simulink model "d2_pacemaker_rate_adaptive"  (R2024b)
settings: Solver=FixedStepAuto  StartTime=0.0  StopTime=10.0  RelTol=1e-3  EnableMultiTasking=on
undefined symbols (not defined in the file): D0, D1, D10, D11, D12, D13, D2, D3, D4, D5, D6, D7, D8, D9, PTA0, PTA1, PTA2, PTB23, PTB9, PTC16, PTC17, PTC2, PTC3, PTC4, PTD0, PTD1, PTD2, PTD3
libraries: frdmk64flib x16, simulink x1
settings Model: ExtModeTrigDuration=5  Creator=cakes  LastModifiedBy=ryans
settings OptimizationCC: EnhancedBackFolding=on  PassReuseOutputArgsAs=Individual arguments  ZeroExternalMemoryAtStartup=off  ZeroInternalMemoryAtStartup=off  MaxStackSize=64  OptimizeBlockOrder=speed  DifferentSizesBufferReuse=on  OptimizationCustomize=off  EfficientTunableParamExpr=on
settings DebuggingCC: ParameterTunabilityLossMsg=error
settings HardwareCC: ProdBitPerPointer=32  ProdBitPerSizeT=32  ProdBitPerPtrDiffT=32  ProdLargestAtomicInteger=Long  ProdLargestAtomicFloat=Double  ProdWordSize=32  ProdHWDeviceType=ARM Compatible->ARM Cortex
settings SFSimCC: MATLABDynamicMemAlloc=off
settings RTWCC: Description=Embedded Coder  SystemTargetFile=ert.tlc  HardwareBoard=NXP FRDM-K64F  TLCOptions="-aInlineSetEventsForThisBaseRateFcn=TLC_FALSE -aSuppressMultiTaskScheduler=TLC_FALSE  -aRateBasedStepFcn=0"  TemplateMakefile=ert_default_tmf  Toolchain=GNU Tools for ARM Embedded Processors  GPUComputeCapability=3.5
settings CodeAppCC: ForceParamTrailComments=on  IgnoreCustomStorageClasses=off  OperatorAnnotations=on  SimulinkDataObjDesc=on  SFDataObjDesc=on  InsertBlockDesc=on
settings ERTTargetCC: ExtModeTransport=4  ExtModeMexFile=sendToCommService  InlinedParameterPlacement=Hierarchical  DynamicArrayContainerType=coder::array

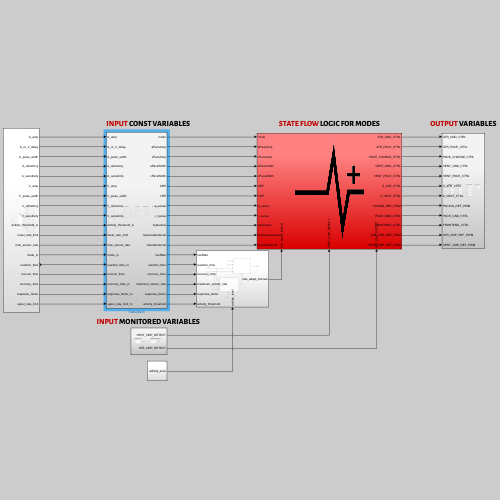
[thumbnail: Simulink's stored preview of the top-level diagram]
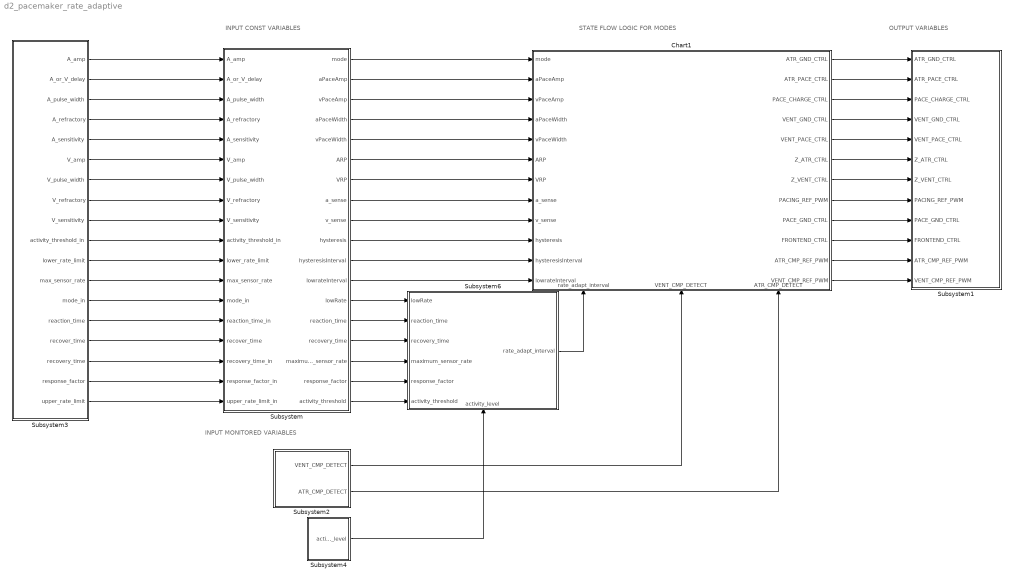
== system d2_pacemaker_rate_adaptive ==
  note: STATE FLOW LOGIC FOR MODES
  note: INPUT CONST VARIABLES
  note: OUTPUT VARIABLES
  note: INPUT MONITORED VARIABLES
  Chart1 : Stateflow chart  TreatAsAtomicUnit=on
      settings: PortSchema="{\"entries\":[{\"content\":{\"sides\":[{\"content\":{\"connectorIds\":[\"In12\",\"In3\",\"In4\",\"In5\",\"In6\",\"In7\",\"In8\",\"In10\",\"In11\",\"In14\",\"In13\",\"In9\"]},\"type\":\"ConnectorPlacement.EquallySpacedRectSide\",\"uuid\":\"0645b224-ea0f-4252-ab3f-59541b69d578\"},{\"content\":{\"connectorIds\":[\"Out1\",\"Out2\",\"Out3\",\"Out4\",\"Out5\",\"Out6\",\"Out7\",\"Out8\",\"Out9\",\"Out10\",\"Out12\",\"Out11\"],\"side\":\"RIGHT\"},\"type\":\"ConnectorPlacement.EquallySpacedRectSide\",\"uuid\":\"774839c9-1eb4-4ab6-be6e-099c2bb8a485\"},{\"content\":{\"side\":\"TOP\"},\"type\":\"ConnectorPlacement.EquallySpacedRectSide\",\"uuid\":\"6cb60565-1780-4b9d-884d-75d2ba8c5024\"},{\"content\":{\"connectorIds\":[\"In15\",\"In1\",\"In2\"],\"side\":\"BOTTOM\"},\"type\":\"ConnectorPlacement.EquallySpacedRectSide\",\"uuid\":\"cb44bc08-16a9-4dba-a42a-7ec56f3e5fd4\"}]},\"type\":\"ConnectorPlacement.EquallySpacedConnector\",\"uuid\":\"755e29d5-bc4e-404e-b866-950d5e4fdc89\"}],\"packageUris\":[\"http://schema.mathworks.com/mf0/Connector/R2020b\"],\"version\":\"1.0\"}"
  Subsystem : Subsystem
  Subsystem1 : Subsystem
  Subsystem2 : Subsystem
  Subsystem3 : Subsystem
  Subsystem4 : Subsystem
  Subsystem6 : Subsystem
      settings: PortSchema="{\"entries\":[{\"content\":{\"sides\":[{\"content\":{\"connectorIds\":[\"In1\",\"In2\",\"In3\",\"In4\",\"In5\",\"In6\"]},\"type\":\"ConnectorPlacement.EquallySpacedRectSide\",\"uuid\":\"7c382d61-8e28-44bb-b5ec-cecd61deb93c\"},{\"content\":{\"connectorIds\":[\"Out1\"],\"side\":\"RIGHT\"},\"type\":\"ConnectorPlacement.EquallySpacedRectSide\",\"uuid\":\"ba607a06-9c8b-48b6-beed-6548638f0809\"},{\"content\":{\"side\":\"TOP\"},\"type\":\"ConnectorPlacement.EquallySpacedRectSide\",\"uuid\":\"ca821f3b-307e-4b9c-9eb8-988783752b3e\"},{\"content\":{\"connectorIds\":[\"In7\"],\"side\":\"BOTTOM\"},\"type\":\"ConnectorPlacement.EquallySpacedRectSide\",\"uuid\":\"dfc7f063-00f5-44f6-92e9-8ee3160489ca\"}]},\"type\":\"ConnectorPlacement.EquallySpacedConnector\",\"uuid\":\"0907d1dd-ec4b-4750-8c68-e4bda9ce45d8\"}],\"packageUris\":[\"http://schema.mathworks.com/mf0/Connector/R2020b\"],\"version\":\"1.0\"}"
  wires:
  Subsystem/2(aPaceAmp) -> Chart1/3(aPaceAmp)
  Subsystem/3(vPaceAmp) -> Chart1/4(vPaceAmp)
  Subsystem/4(aPaceWidth) -> Chart1/5(aPaceWidth)
  Subsystem/5(vPaceWidth) -> Chart1/6(vPaceWidth)
  Subsystem/6(ARP) -> Chart1/7(ARP)
  Subsystem/7(VRP) -> Chart1/8(VRP)
  Subsystem/12(lowrateInterval) -> Chart1/9(lowrateInterval)
  Subsystem/1(mode) -> Chart1/12(mode)
  Chart1/1(ATR_GND_CTRL) -> Subsystem1/1(ATR_GND_CTRL)
  Chart1/2(ATR_PACE_CTRL) -> Subsystem1/2(ATR_PACE_CTRL)
  Chart1/3(PACE_CHARGE_CTRL) -> Subsystem1/3(PACE_CHARGE_CTRL)
  Chart1/4(VENT_GND_CTRL) -> Subsystem1/4(VENT_GND_CTRL)
  Chart1/5(VENT_PACE_CTRL) -> Subsystem1/5(VENT_PACE_CTRL)
  Chart1/6(Z_ATR_CTRL) -> Subsystem1/6(Z_ATR_CTRL)
  Subsystem2/1(VENT_CMP_DETECT) -> Chart1/1(VENT_CMP_DETECT)
  Chart1/9(PACE_GND_CTRL) -> Subsystem1/9(PACE_GND_CTRL)
  Subsystem/8(a_sense) -> Chart1/10(a_sense)
  Subsystem/9(v_sense) -> Chart1/11(v_sense)
  Chart1/10(FRONTEND_CTRL) -> Subsystem1/10(FRONTEND_CTRL)
  Chart1/11(VENT_CMP_REF_PWM) -> Subsystem1/12(VENT_CMP_REF_PWM)
  Chart1/7(Z_VENT_CTRL) -> Subsystem1/7(Z_VENT_CTRL)
  Chart1/8(PACING_REF_PWM) -> Subsystem1/8(PACING_REF_PWM)
  Chart1/12(ATR_CMP_REF_PWM) -> Subsystem1/11(ATR_CMP_REF_PWM)
  Subsystem2/2(ATR_CMP_DETECT) -> Chart1/2(ATR_CMP_DETECT)
  Subsystem/10(hysteresis) -> Chart1/14(hysteresis)
  Subsystem/11(hysteresisInterval) -> Chart1/13(hysteresisInterval)
  Subsystem/17(response_factor) -> Subsystem6/5(response_factor)
  Subsystem/16(maximum_sensor_rate) -> Subsystem6/4(maximum_sensor_rate)
  Subsystem/13(lowRate) -> Subsystem6/1(lowRate)
  Subsystem/14(reaction_time) -> Subsystem6/2(reaction_time)
  Subsystem/15(recovery_time) -> Subsystem6/3(recovery_time)
  Subsystem/18(activity_threshold) -> Subsystem6/6(activity_threshold)
  Subsystem6/1(rate_adapt_interval) -> Chart1/15(rate_adapt_interval)
  Subsystem4/1(activity_level) -> Subsystem6/7(activity_level)
  Subsystem3/1(A_amp) -> Subsystem/1(A_amp)
  Subsystem3/3(A_pulse_width) -> Subsystem/3(A_pulse_width)
  Subsystem3/4(A_refractory) -> Subsystem/4(A_refractory)
  Subsystem3/5(A_sensitivity) -> Subsystem/5(A_sensitivity)
  Subsystem3/6(V_amp) -> Subsystem/6(V_amp)
  Subsystem3/7(V_pulse_width) -> Subsystem/7(V_pulse_width)
  Subsystem3/8(V_refractory) -> Subsystem/8(V_refractory)
  Subsystem3/9(V_sensitivity) -> Subsystem/9(V_sensitivity)
  Subsystem3/11(lower_rate_limit) -> Subsystem/11(lower_rate_limit)
  Subsystem3/12(max_sensor_rate) -> Subsystem/12(max_sensor_rate)
  Subsystem3/13(mode_in) -> Subsystem/13(mode_in)
  Subsystem3/15(recover_time) -> Subsystem/15(recover_time)
  Subsystem3/16(recovery_time) -> Subsystem/16(recovery_time_in)
  Subsystem3/17(response_factor) -> Subsystem/17(response_factor_in)
  Subsystem3/18(upper_rate_limit) -> Subsystem/18(upper_rate_limit_in)
  Subsystem3/2(A_or_V_delay) -> Subsystem/2(A_or_V_delay)
  Subsystem3/10(activity_threshold_in) -> Subsystem/10(activity_threshold_in)
  Subsystem3/14(reaction_time) -> Subsystem/14(reaction_time_in)

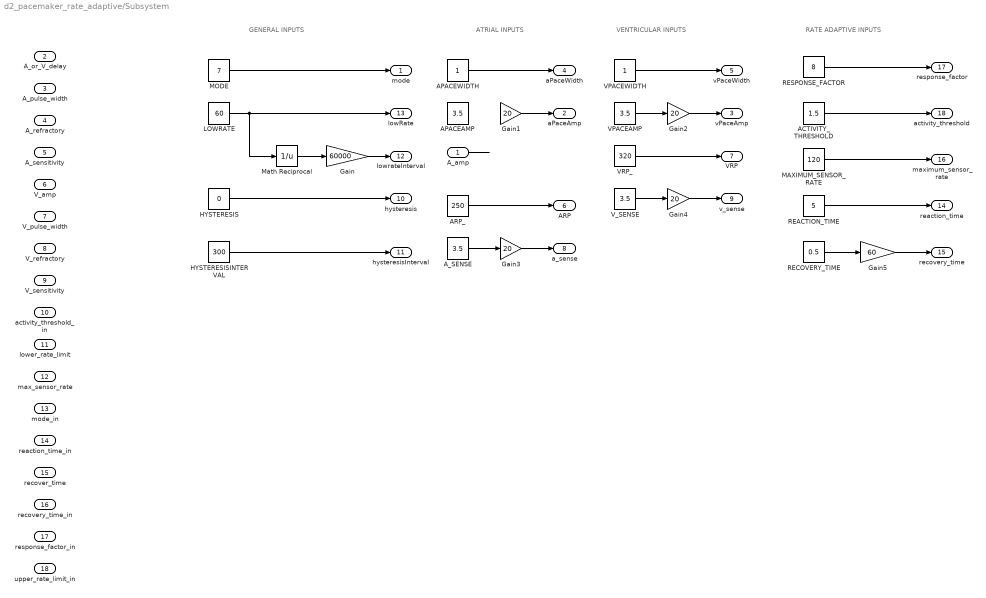
== system d2_pacemaker_rate_adaptive/Subsystem ==
  note: GENERAL INPUTS
  note: ATRIAL INPUTS
  note: VENTRICULAR INPUTS
  note: RATE ADAPTIVE INPUTS
  A_amp : Inport  OutDataTypeStr=single
  A_or_V_delay : Inport  Port=2
  A_pulse_width : Inport  Port=3
  A_refractory : Inport  Port=4
  A_sensitivity : Inport  Port=5
  V_amp : Inport  Port=6
  V_pulse_width : Inport  Port=7
  V_refractory : Inport  Port=8
  V_sensitivity : Inport  Port=9
  activity_threshold_in : Inport  Port=10
  lower_rate_limit : Inport  Port=11
  max_sensor_rate : Inport  Port=12
  mode_in : Inport  Port=13
  reaction_time_in : Inport  Port=14
  recover_time : Inport  Port=15
  recovery_time_in : Inport  Port=16
  response_factor_in : Inport  Port=17
  upper_rate_limit_in : Inport  Port=18
  ACTIVITY_THRESHOLD : Constant  Value=1.5
  APACEAMP : Constant  Value=3.5
  APACEWIDTH : Constant
  ARP_ : Constant  Value=250
  A_SENSE : Constant  Value=3.5
  Gain : Gain  Gain=60000
  Gain{1..4} (4 alike) : Gain  Gain=20
  Gain5 : Gain  Gain=60
  HYSTERESIS : Constant  Value=0
  HYSTERESISINTERVAL : Constant  Value=300
  LOWRATE : Constant  Value=60
  MAXIMUM_SENSOR_RATE : Constant  Value=120
  MODE : Constant  Value=7
  Math Reciprocal : Math  Operator=reciprocal  SignedPower=on
  REACTION_TIME : Constant  Value=5
  RECOVERY_TIME : Constant  Value=0.5
  RESPONSE_FACTOR : Constant  Value=8
  VPACEAMP : Constant  Value=3.5
  VPACEWIDTH : Constant
  VRP_ : Constant  Value=320
  V_SENSE : Constant  Value=3.5
  mode : Outport
  aPaceAmp : Outport  Port=2
  vPaceAmp : Outport  Port=3
  aPaceWidth : Outport  Port=4
  vPaceWidth : Outport  Port=5
  ARP : Outport  Port=6
  VRP : Outport  Port=7
  a_sense : Outport  Port=8
  v_sense : Outport  Port=9
  hysteresis : Outport  Port=10
  hysteresisInterval : Outport  Port=11
  lowrateInterval : Outport  Port=12
  lowRate : Outport  Port=13
  reaction_time : Outport  Port=14
  recovery_time : Outport  Port=15
  maximum_sensor_rate : Outport  Port=16
  response_factor : Outport  Port=17
  activity_threshold : Outport  Port=18
  wires:
  APACEWIDTH/1 -> aPaceWidth/1
  VPACEWIDTH/1 -> vPaceWidth/1
  MODE/1 -> mode/1
  ARP_/1 -> ARP/1
  VRP_/1 -> VRP/1
  HYSTERESIS/1 -> hysteresis/1
  HYSTERESISINTERVAL/1 -> hysteresisInterval/1
  LOWRATE/1 -> lowRate/1, Math Reciprocal/1
  Math Reciprocal/1 -> Gain/1
  Gain/1 -> lowrateInterval/1
  Gain1/1 -> aPaceAmp/1
  VPACEAMP/1 -> Gain2/1
  Gain2/1 -> vPaceAmp/1
  A_SENSE/1 -> Gain3/1
  V_SENSE/1 -> Gain4/1
  Gain4/1 -> v_sense/1
  Gain3/1 -> a_sense/1
  RESPONSE_FACTOR/1 -> response_factor/1
  ACTIVITY_THRESHOLD/1 -> activity_threshold/1
  RECOVERY_TIME/1 -> Gain5/1
  Gain5/1 -> recovery_time/1
  REACTION_TIME/1 -> reaction_time/1
  MAXIMUM_SENSOR_RATE/1 -> maximum_sensor_rate/1
  A_amp/1 -> ?

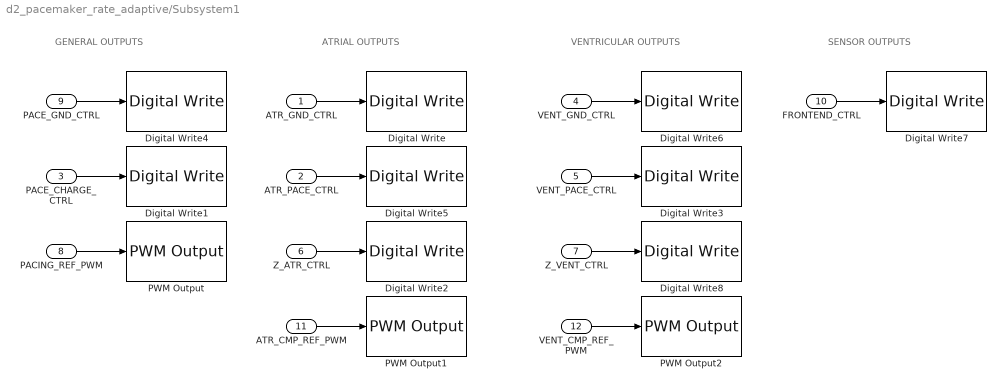
== system d2_pacemaker_rate_adaptive/Subsystem1 ==
  note: ATRIAL OUTPUTS
  note: GENERAL OUTPUTS
  note: VENTRICULAR OUTPUTS
  note: SENSOR OUTPUTS
  ATR_GND_CTRL : Inport
  ATR_PACE_CTRL : Inport  Port=2
  PACE_CHARGE_CTRL : Inport  Port=3
  VENT_GND_CTRL : Inport  Port=4
  VENT_PACE_CTRL : Inport  Port=5
  Z_ATR_CTRL : Inport  Port=6
  Z_VENT_CTRL : Inport  Port=7
  PACING_REF_PWM : Inport  Port=8
  PACE_GND_CTRL : Inport  Port=9
  FRONTEND_CTRL : Inport  Port=10
  ATR_CMP_REF_PWM : Inport  Port=11
  VENT_CMP_REF_PWM : Inport  Port=12
  Digital Write : frdmk64flib/Digital Write  Whichpin=PTD2 (D11)
  Digital Write1 : frdmk64flib/Digital Write  Whichpin=PTB9 (D2)
  Digital Write2 : frdmk64flib/Digital Write  Whichpin=PTB23 (D4)
  Digital Write3 : frdmk64flib/Digital Write  Whichpin=PTC4 (D9)
  Digital Write4 : frdmk64flib/Digital Write  Whichpin=PTD0 (D10)
  Digital Write5 : frdmk64flib/Digital Write  Whichpin=PTA0 (D8)
  Digital Write6 : frdmk64flib/Digital Write  Whichpin=PTD3 (D12)
  Digital Write7 : frdmk64flib/Digital Write  Whichpin=PTD1 (D13)
  Digital Write8 : frdmk64flib/Digital Write  Whichpin=PTC3 (D7)
  PWM Output : frdmk64flib/PWM Output  Whichpin=PTA2 (D5)  InitialFrequency=2000  InitialDutyCycle=0
  PWM Output1 : frdmk64flib/PWM Output  Whichpin=PTC2 (D6)  InitialFrequency=2000  InitialDutyCycle=0
  PWM Output2 : frdmk64flib/PWM Output  Whichpin=PTA1 (D3)  InitialFrequency=2000  InitialDutyCycle=0
  wires:
  PACING_REF_PWM/1 -> PWM Output/1
  Z_ATR_CTRL/1 -> Digital Write2/1
  PACE_CHARGE_CTRL/1 -> Digital Write1/1
  ATR_PACE_CTRL/1 -> Digital Write5/1
  ATR_GND_CTRL/1 -> Digital Write/1
  VENT_PACE_CTRL/1 -> Digital Write3/1
  VENT_GND_CTRL/1 -> Digital Write6/1
  FRONTEND_CTRL/1 -> Digital Write7/1
  Z_VENT_CTRL/1 -> Digital Write8/1
  PACE_GND_CTRL/1 -> Digital Write4/1
  ATR_CMP_REF_PWM/1 -> PWM Output1/1
  VENT_CMP_REF_PWM/1 -> PWM Output2/1

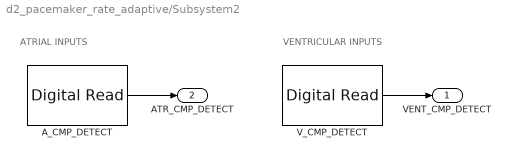
== system d2_pacemaker_rate_adaptive/Subsystem2 ==
  note: ATRIAL INPUTS
  note: VENTRICULAR INPUTS
  A_CMP_DETECT : frdmk64flib/Digital Read  Whichpin=PTC16 (D0)  SampleTime=0.01
  V_CMP_DETECT : frdmk64flib/Digital Read  Whichpin=PTC17 (D1)  SampleTime=0.01
  VENT_CMP_DETECT : Outport
  ATR_CMP_DETECT : Outport  Port=2
  wires:
  V_CMP_DETECT/1 -> VENT_CMP_DETECT/1
  A_CMP_DETECT/1 -> ATR_CMP_DETECT/1

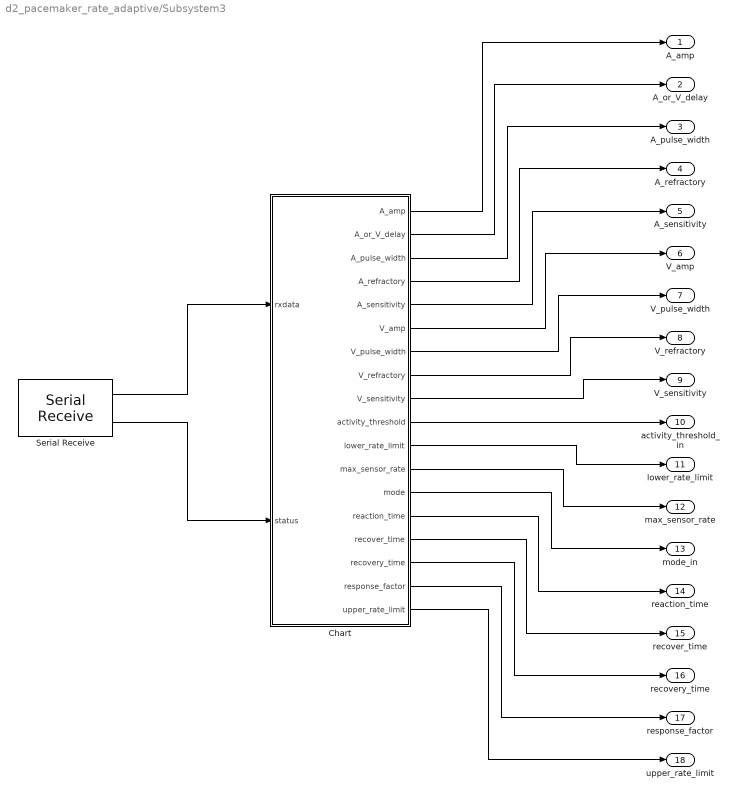
== system d2_pacemaker_rate_adaptive/Subsystem3 ==
  Chart : Stateflow chart  TreatAsAtomicUnit=on
  Serial Receive : frdmk64flib/Serial Receive  SCIModule=0  Baudrate=uint32(9600)  Parity=None  StopBits=1  HardwareFlowControl=None  ByteOrder=LittleEndian  DataType=uint8  DataLength=10  BlockingMode=off  OutputStatus=on  SampleTime=0.1
  A_amp : Outport
  A_or_V_delay : Outport  Port=2
  A_pulse_width : Outport  Port=3
  A_refractory : Outport  Port=4
  A_sensitivity : Outport  Port=5
  V_amp : Outport  Port=6
  V_pulse_width : Outport  Port=7
  V_refractory : Outport  Port=8
  V_sensitivity : Outport  Port=9
  activity_threshold_in : Outport  Port=10
  lower_rate_limit : Outport  Port=11
  max_sensor_rate : Outport  Port=12
  mode_in : Outport  Port=13
  reaction_time : Outport  Port=14
  recover_time : Outport  Port=15
  recovery_time : Outport  Port=16
  response_factor : Outport  Port=17
  upper_rate_limit : Outport  Port=18
  wires:
  Serial Receive/1 -> Chart/1(rxdata)
  Serial Receive/2 -> Chart/2(status)
  Chart/1(A_amp) -> A_amp/1
  Chart/2(A_or_V_delay) -> A_or_V_delay/1
  Chart/3(A_pulse_width) -> A_pulse_width/1
  Chart/4(A_refractory) -> A_refractory/1
  Chart/5(A_sensitivity) -> A_sensitivity/1
  Chart/6(V_amp) -> V_amp/1
  Chart/7(V_pulse_width) -> V_pulse_width/1
  Chart/8(V_refractory) -> V_refractory/1
  Chart/9(V_sensitivity) -> V_sensitivity/1
  Chart/10(activity_threshold) -> activity_threshold_in/1
  Chart/11(lower_rate_limit) -> lower_rate_limit/1
  Chart/12(max_sensor_rate) -> max_sensor_rate/1
  Chart/13(mode) -> mode_in/1
  Chart/14(reaction_time) -> reaction_time/1
  Chart/15(recover_time) -> recover_time/1
  Chart/16(recovery_time) -> recovery_time/1
  Chart/17(response_factor) -> response_factor/1
  Chart/18(upper_rate_limit) -> upper_rate_limit/1

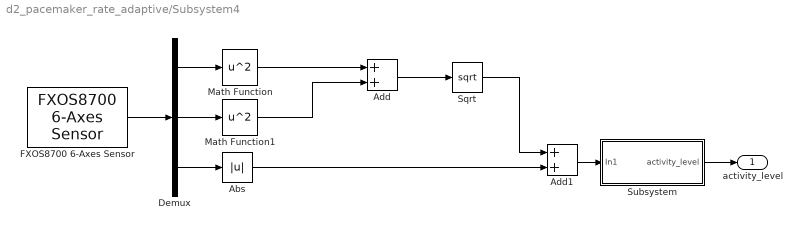
== system d2_pacemaker_rate_adaptive/Subsystem4 ==
  Abs : Abs  SaturateOnIntegerOverflow=off
  Add : Sum
  Add1 : Sum
  Demux : Demux  Outputs=3
  FXOS8700 6-Axes Sensor : frdmk64flib/FXOS8700 6-Axes Sensor  Activesensor=Accelerometer only  ODR=50Hz  HybridODR=400Hz  Accelfullrange=-4g to +4g  SampleTime=0.01
  Math Function : Math  Operator=square
  Math Function1 : Math  Operator=square
  Sqrt : Sqrt
  Subsystem : Subsystem
  activity_level : Outport
  wires:
  Demux/2 -> Math Function1/1
  Math Function/1 -> Add/1
  Math Function1/1 -> Add/2
  Sqrt/1 -> Add1/1
  Abs/1 -> Add1/2
  Add/1 -> Sqrt/1
  Demux/1 -> Math Function/1
  Demux/3 -> Abs/1
  FXOS8700 6-Axes Sensor/1 -> Demux/1
  Add1/1 -> Subsystem/1(In1)
  Subsystem/1(activity_level) -> activity_level/1

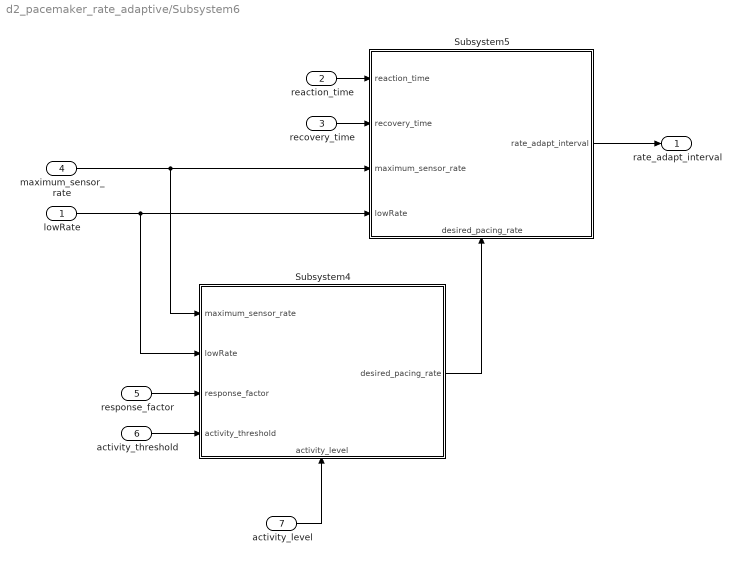
== system d2_pacemaker_rate_adaptive/Subsystem6 ==
  lowRate : Inport
  reaction_time : Inport  Port=2
  recovery_time : Inport  Port=3
  maximum_sensor_rate : Inport  Port=4
  response_factor : Inport  Port=5
  activity_threshold : Inport  Port=6
  activity_level : Inport  Port=7
  Subsystem4 : Subsystem
      settings: PortSchema="{\"entries\":[{\"content\":{\"sides\":[{\"content\":{\"connectorIds\":[\"In1\",\"In2\",\"In3\",\"In4\"]},\"type\":\"ConnectorPlacement.EquallySpacedRectSide\",\"uuid\":\"79bc3fb3-9fea-4441-ae48-8f2cb8dc5d6d\"},{\"content\":{\"connectorIds\":[\"Out1\"],\"side\":\"RIGHT\"},\"type\":\"ConnectorPlacement.EquallySpacedRectSide\",\"uuid\":\"8e25f63d-7a7f-4a30-9d51-ff4e93a9aa99\"},{\"content\":{\"side\":\"TOP\"},\"type\":\"ConnectorPlacement.EquallySpacedRectSide\",\"uuid\":\"e07be596-e475-4181-9b08-2e1f9ea03076\"},{\"content\":{\"connectorIds\":[\"In5\"],\"side\":\"BOTTOM\"},\"type\":\"ConnectorPlacement.EquallySpacedRectSide\",\"uuid\":\"45319594-5d17-4fc8-9d4a-dc1aca31fcf6\"}]},\"type\":\"ConnectorPlacement.EquallySpacedConnector\",\"uuid\":\"3beff34e-2a6c-47b3-9523-1069d662617f\"}],\"packageUris\":[\"http://schema.mathworks.com/mf0/Connector/R2020b\"],\"version\":\"1.0\"}"
  Subsystem5 : Subsystem
      settings: PortSchema="{\"entries\":[{\"content\":{\"sides\":[{\"content\":{\"connectorIds\":[\"In1\",\"In2\",\"In3\",\"In4\"]},\"type\":\"ConnectorPlacement.EquallySpacedRectSide\",\"uuid\":\"79bc3fb3-9fea-4441-ae48-8f2cb8dc5d6d\"},{\"content\":{\"connectorIds\":[\"Out1\"],\"side\":\"RIGHT\"},\"type\":\"ConnectorPlacement.EquallySpacedRectSide\",\"uuid\":\"8e25f63d-7a7f-4a30-9d51-ff4e93a9aa99\"},{\"content\":{\"side\":\"TOP\"},\"type\":\"ConnectorPlacement.EquallySpacedRectSide\",\"uuid\":\"e07be596-e475-4181-9b08-2e1f9ea03076\"},{\"content\":{\"connectorIds\":[\"In5\"],\"side\":\"BOTTOM\"},\"type\":\"ConnectorPlacement.EquallySpacedRectSide\",\"uuid\":\"37a509d1-15c0-445b-9b56-eefd17d0fdfa\"}]},\"type\":\"ConnectorPlacement.EquallySpacedConnector\",\"uuid\":\"3beff34e-2a6c-47b3-9523-1069d662617f\"}],\"packageUris\":[\"http://schema.mathworks.com/mf0/Connector/R2020b\"],\"version\":\"1.0\"}"
  rate_adapt_interval : Outport
  wires:
  Subsystem5/1(rate_adapt_interval) -> rate_adapt_interval/1
  reaction_time/1 -> Subsystem5/1(reaction_time)
  recovery_time/1 -> Subsystem5/2(recovery_time)
  Subsystem4/1(desired_pacing_rate) -> Subsystem5/5(desired_pacing_rate)
  maximum_sensor_rate/1 -> Subsystem4/1(maximum_sensor_rate), Subsystem5/3(maximum_sensor_rate)
  lowRate/1 -> Subsystem4/2(lowRate), Subsystem5/4(lowRate)
  activity_threshold/1 -> Subsystem4/4(activity_threshold)
  response_factor/1 -> Subsystem4/3(response_factor)
  activity_level/1 -> Subsystem4/5(activity_level)

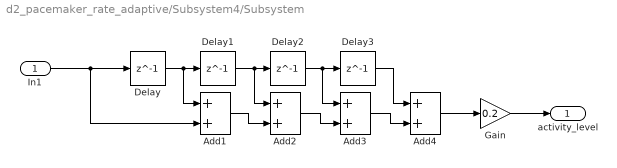
== system d2_pacemaker_rate_adaptive/Subsystem4/Subsystem ==
  In1 : Inport
  Add{1..4} (4 alike) : Sum
  Delay{,1..3} (4 alike) : Delay  DelayLength=1
  Gain : Gain  Gain=0.2
  activity_level : Outport
  wires:
  Delay/1 -> Add1/1, Delay1/1
  Delay1/1 -> Add2/1, Delay2/1
  Delay2/1 -> Add3/1, Delay3/1
  In1/1 -> Delay/1, Add1/2
  Add1/1 -> Add2/2
  Add4/1 -> Gain/1
  Add2/1 -> Add3/2
  Add3/1 -> Add4/2
  Delay3/1 -> Add4/1
  Gain/1 -> activity_level/1

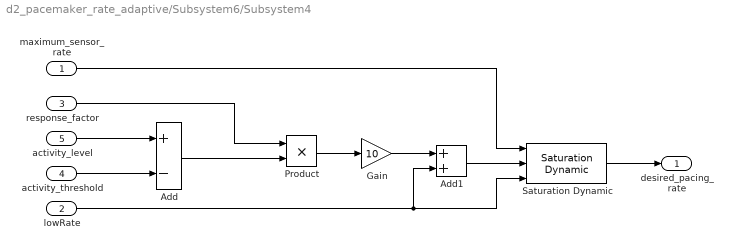
== system d2_pacemaker_rate_adaptive/Subsystem6/Subsystem4 ==
  maximum_sensor_rate : Inport
  lowRate : Inport  Port=2
  response_factor : Inport  Port=3
  activity_threshold : Inport  Port=4
  activity_level : Inport  Port=5
  Add : Sum  Inputs=+-
  Add1 : Sum
  Gain : Gain  Gain=10
  Product : Product
  Saturation Dynamic : simulink/Discontinuities/Saturation Dynamic  OutMin=[]  OutMax=[]  OutDataTypeStr=Inherit: Same as second input  OutDataType=fixdt(1, 16)  OutScaling=2^-10  DoSatur=off
  desired_pacing_rate : Outport
  wires:
  activity_level/1 -> Add/1
  activity_threshold/1 -> Add/2
  Add/1 -> Product/2
  response_factor/1 -> Product/1
  Gain/1 -> Add1/1
  Product/1 -> Gain/1
  lowRate/1 -> Saturation Dynamic/3, Add1/2
  Add1/1 -> Saturation Dynamic/2
  maximum_sensor_rate/1 -> Saturation Dynamic/1
  Saturation Dynamic/1 -> desired_pacing_rate/1

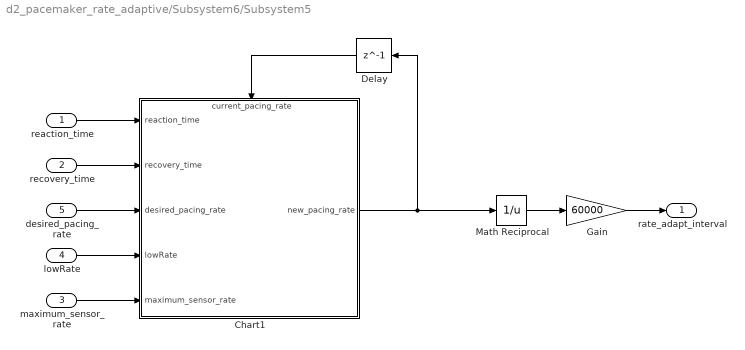
== system d2_pacemaker_rate_adaptive/Subsystem6/Subsystem5 ==
  reaction_time : Inport
  recovery_time : Inport  Port=2
  maximum_sensor_rate : Inport  Port=3
  lowRate : Inport  Port=4
  desired_pacing_rate : Inport  Port=5
  Chart1 : Stateflow chart  TreatAsAtomicUnit=on
      settings: PortSchema="{\"entries\":[{\"content\":{\"sides\":[{\"content\":{\"connectorIds\":[\"In2\",\"In3\",\"In4\",\"In5\",\"In6\"]},\"type\":\"ConnectorPlacement.EquallySpacedRectSide\",\"uuid\":\"06a0217b-4288-43b0-8932-705b4d4ece1e\"},{\"content\":{\"connectorIds\":[\"Out1\"],\"side\":\"RIGHT\"},\"type\":\"ConnectorPlacement.EquallySpacedRectSide\",\"uuid\":\"c8eefe2e-d095-40c8-acb0-aebaf19a9365\"},{\"content\":{\"connectorIds\":[\"In1\"],\"side\":\"TOP\"},\"type\":\"ConnectorPlacement.EquallySpacedRectSide\",\"uuid\":\"128ffed5-e0e5-4f4f-9131-f15ad41e2462\"},{\"content\":{\"side\":\"BOTTOM\"},\"type\":\"ConnectorPlacement.EquallySpacedRectSide\",\"uuid\":\"a7475944-bf84-45a0-8219-ddf2a50d7d23\"}]},\"type\":\"ConnectorPlacement.EquallySpacedConnector\",\"uuid\":\"00626f3d-df19-4fc7-9d9d-9a6ae210b908\"}],\"packageUris\":[\"http://schema.mathworks.com/mf0/Connector/R2020b\"],\"version\":\"1.0\"}"
  Delay : Delay  DelayLength=1  InitialCondition=0
  Gain : Gain  Gain=60000
  Math Reciprocal : Math  Operator=reciprocal  SignedPower=on
  rate_adapt_interval : Outport
  wires:
  Chart1/1(new_pacing_rate) -> Delay/1, Math Reciprocal/1
  Math Reciprocal/1 -> Gain/1
  Gain/1 -> rate_adapt_interval/1
  reaction_time/1 -> Chart1/2(reaction_time)
  Delay/1 -> Chart1/1(current_pacing_rate)
  maximum_sensor_rate/1 -> Chart1/6(maximum_sensor_rate)
  recovery_time/1 -> Chart1/3(recovery_time)
  lowRate/1 -> Chart1/5(lowRate)
  desired_pacing_rate/1 -> Chart1/4(desired_pacing_rate)

== stateflow chart d2_pacemaker_rate_adaptive/Chart1 ==
  settings: sampleTime=0.001
  state INIT
    entry:
    %inital state, reset variables when mode change
    PACE_CHARGE_CTRL = 0;
    ATR_PACE_CTRL = 0;
    ATR_GND_CTRL = 0;
    VENT_PACE_CTRL=0;
    VENT_GND_CTRL=0;
    Z_ATR_CTRL = 0;
    Z_VENT_CTRL=0;
    PACE_GND_CTRL=0;
    PACING_REF_PWM=0;
    PACE_CHARGE_CTRL=0;
    FRONTEND_CTRL =0;
    VENT_CMP_REF_PWM = v_sense;
    ATR_CMP_REF_PWM = a_sense;
    note: MODE
        | NUMBER
        |
        | AOO
        | 0
        |
        | VOO
        | 1
        |
        | AAI
        | 2
        |
        | VVI
        | 3
  state AOO
    state AOO_Charging
      %charging capacitor
      entry:
      PACING_REF_PWM = aPaceAmp;
      PACE_GND_CTRL = 1;
      Z_ATR_CTRL = 0;
      ATR_PACE_CTRL = 0;
      PACE_CHARGE_CTRL = 1;
      ATR_GND_CTRL = 1;
    state AOO_Pacing
      %discharging
      entry:
      Z_ATR_CTRL = 1;
      PACE_CHARGE_CTRL = 0;
      ATR_GND_CTRL = 0;
      ATR_PACE_CTRL = 1;
    (default) -> AOO_Charging
    AOO_Charging -> AOO_Pacing : after(lowrateInterval - aPaceWidth, msec)
    AOO_Pacing -> AOO_Charging : after(aPaceWidth, msec)
  state VOO
    state VOO_Charging
      %charging capacitor
      entry:
      PACING_REF_PWM = vPaceAmp;
      PACE_GND_CTRL = 1;
      Z_VENT_CTRL = 0;
      VENT_PACE_CTRL = 0;
      PACE_CHARGE_CTRL = 1;
      VENT_GND_CTRL = 1;
    state VOO_Pacing
      %discharging capacitor
      entry:
      Z_VENT_CTRL = 1;
      PACE_CHARGE_CTRL = 0;
      VENT_GND_CTRL = 0;
      VENT_PACE_CTRL = 1;
    (default) -> VOO_Charging
    VOO_Charging -> VOO_Pacing : after(lowrateInterval - vPaceWidth, msec)
    VOO_Pacing -> VOO_Charging : after(vPaceWidth, msec)
  state AAI
    state pARP
      %atrial refractory period from paced beat
      entry:
      FRONTEND_CTRL = 1;
      PACING_REF_PWM = aPaceAmp;
      PACE_GND_CTRL=1;
      ATR_PACE_CTRL = 0;
      PACE_CHARGE_CTRL = 1;
      ATR_GND_CTRL = 1;
    state pReady
      %refratory period
      %finishes after
      %paced beat
    state Discharging
      %discharging
      entry:
      PACE_CHARGE_CTRL = 0;
      ATR_GND_CTRL = 0;
      ATR_PACE_CTRL = 1;
    state sARP
      %atrial refractory
      %period from
      %sensed beat
    state sReady
      %refratory period
      %finishes after
      %sensed beat
    AAI.Discharging -> AAI.pARP : after(aPaceWidth, msec)
    (default) -> AAI.pARP
    AAI.pARP -> AAI.pReady : after(ARP,  msec)
    AAI.pReady -> AAI.Discharging [order 1] : after(lowrateInterval - ARP - aPaceWidth, msec)
    AAI.pReady -> AAI.sARP [order 2] : [ATR_CMP_DETECT]
    AAI.sReady -> AAI.Discharging [order 1] : after(lowrateInterval - ARP- aPaceWidth + (hysteresis * hysteresisInterval), msec)
    AAI.sARP -> AAI.sReady : after(ARP, msec)
    AAI.sReady -> AAI.sARP [order 2] : [ATR_CMP_DETECT]
  state VVI
    state pVRP
      %ventricular refractory period from paced beat
      entry:
      FRONTEND_CTRL = 1;
      PACING_REF_PWM = vPaceAmp;
      PACE_GND_CTRL=1;
      VENT_PACE_CTRL = 0;
      PACE_CHARGE_CTRL = 1;
      VENT_GND_CTRL = 1;
    state pReady
      %refratory period
      %finishes after
      %paced beat
    state Discharging
      %discharging
      entry:
      PACE_CHARGE_CTRL = 0;
      VENT_GND_CTRL = 0;
      VENT_PACE_CTRL = 1;
    state sVRP
      %atrial refractory
      %period from
      %sensed beat
    state sReady
      %refratory period
      %finishes after
      %sensed beat
    VVI.Discharging -> VVI.pVRP : after(vPaceWidth, msec)
    (default) -> VVI.pVRP
    VVI.pVRP -> VVI.pReady : after(VRP, msec)
    VVI.pReady -> VVI.Discharging [order 1] : after(lowrateInterval - VRP - vPaceWidth, msec)
    VVI.pReady -> VVI.sVRP [order 2] : [VENT_CMP_DETECT]
    VVI.sReady -> VVI.Discharging [order 1] : after(lowrateInterval - VRP - vPaceWidth + (hysteresis * hysteresisInterval), msec)
    VVI.sVRP -> VVI.sReady : after(VRP, msec)
    VVI.sReady -> VVI.sVRP [order 2] : [VENT_CMP_DETECT]
  state AOOR
    state AOOR_Charging
      %charging capacitor
      entry:
      PACING_REF_PWM = aPaceAmp;
      PACE_GND_CTRL = 1;
      Z_ATR_CTRL = 0;
      ATR_PACE_CTRL = 0;
      PACE_CHARGE_CTRL = 1;
      ATR_GND_CTRL = 1;
    state AOOR_Pacing
      %discharging
      entry:
      Z_ATR_CTRL = 1;
      PACE_CHARGE_CTRL = 0;
      ATR_GND_CTRL = 0;
      ATR_PACE_CTRL = 1;
    (default) -> AOOR_Charging
    AOOR_Charging -> AOOR_Pacing : after(rate_adapt_interval - aPaceWidth, msec)
    AOOR_Pacing -> AOOR_Charging : after(aPaceWidth, msec)
  state VOOR
    state VOOR_Charging
      %charging capacitor
      entry:
      PACING_REF_PWM = vPaceAmp;
      PACE_GND_CTRL = 1;
      Z_VENT_CTRL = 0;
      VENT_PACE_CTRL = 0;
      PACE_CHARGE_CTRL = 1;
      VENT_GND_CTRL = 1;
    state VOOR_Pacing
      %discharging capacitor
      entry:
      Z_VENT_CTRL = 1;
      PACE_CHARGE_CTRL = 0;
      VENT_GND_CTRL = 0;
      VENT_PACE_CTRL = 1;
    (default) -> VOOR_Charging
    VOOR_Charging -> VOOR_Pacing : after(rate_adapt_interval - vPaceWidth, msec)
    VOOR_Pacing -> VOOR_Charging : after(vPaceWidth,msec)
  state AAIR
    state pARP
      %atrial refractory period from paced beat
      entry:
      FRONTEND_CTRL = 1;
      PACING_REF_PWM = aPaceAmp;
      PACE_GND_CTRL=1;
      ATR_PACE_CTRL = 0;
      PACE_CHARGE_CTRL = 1;
      ATR_GND_CTRL = 1;
    state pReady
      %refratory period
      %finishes after
      %paced beat
    state Discharging
      %discharging
      entry:
      PACE_CHARGE_CTRL = 0;
      ATR_GND_CTRL = 0;
      ATR_PACE_CTRL = 1;
    state sARP
      %atrial refractory
      %period from
      %sensed beat
    state sReady
      %refratory period
      %finishes after
      %sensed beat
    AAIR.Discharging -> AAIR.pARP : after(aPaceWidth, msec)
    (default) -> AAIR.pARP
    AAIR.pARP -> AAIR.pReady : after(ARP,  msec)
    AAIR.pReady -> AAIR.Discharging [order 1] : after(rate_adapt_interval - ARP - aPaceWidth, msec)
    AAIR.pReady -> AAIR.sARP [order 2] : [ATR_CMP_DETECT]
    AAIR.sReady -> AAIR.Discharging [order 1] : after(rate_adapt_interval - ARP- aPaceWidth + (hysteresis * hysteresisInterval), msec)
    AAIR.sARP -> AAIR.sReady : after(ARP, msec)
    AAIR.sReady -> AAIR.sARP [order 2] : [ATR_CMP_DETECT]
  state VVIR
    state pVRP
      %ventricular refractory period from paced beat
      entry:
      FRONTEND_CTRL = 1;
      PACING_REF_PWM = vPaceAmp;
      PACE_GND_CTRL=1;
      VENT_PACE_CTRL = 0;
      PACE_CHARGE_CTRL = 1;
      VENT_GND_CTRL = 1;
    state pReady
      %refratory period
      %finishes after
      %paced beat
    state Discharging
      %discharging
      entry:
      PACE_CHARGE_CTRL = 0;
      VENT_GND_CTRL = 0;
      VENT_PACE_CTRL = 1;
    state sVRP
      %atrial refractory
      %period from
      %sensed beat
    state sReady
      %refratory period
      %finishes after
      %sensed beat
    VVIR.Discharging -> VVIR.pVRP : after(vPaceWidth, msec)
    (default) -> VVIR.pVRP
    VVIR.pVRP -> VVIR.pReady : after(VRP, msec)
    VVIR.pReady -> VVIR.Discharging [order 1] : after(rate_adapt_interval - VRP - vPaceWidth, msec)
    VVIR.pReady -> VVIR.sVRP [order 2] : [VENT_CMP_DETECT]
    VVIR.sReady -> VVIR.Discharging [order 1] : after(rate_adapt_interval - VRP - vPaceWidth + (hysteresis * hysteresisInterval), msec)
    VVIR.sVRP -> VVIR.sReady : after(VRP, msec)
    VVIR.sReady -> VVIR.sVRP [order 2] : [VENT_CMP_DETECT]
  INIT -> AOO [order 1] : [mode == 0]
  AOO -> INIT : [mode ~=0]
  INIT -> VOO [order 2] : [mode==1]
  VOO -> INIT : [mode~=1]
  INIT -> AAI [order 3] : [mode == 2]
  AAI -> INIT : [mode ~=2]
  INIT -> VVI [order 4] : [mode==3]
  VVI -> INIT : [mode~=3]
  INIT -> AOOR [order 5] : [mode==4]
  AOOR -> INIT : [mode~=4]
  (default) -> INIT
  INIT -> VOOR [order 6] : [mode==5]
  VOOR -> INIT : [mode~=5]
  INIT -> AAIR [order 7] : [mode==6]
  AAIR -> INIT : [mode~=6]
  INIT -> VVIR [order 8] : [mode==7]
  VVIR -> INIT : [mode~=7]
  data: VENT_CMP_DETECT input; ATR_CMP_DETECT input; ATR_GND_CTRL output; ATR_PACE_CTRL output; PACE_CHARGE_CTRL output; VENT_GND_CTRL output; VENT_PACE_CTRL output; Z_ATR_CTRL output; aPaceAmp input; vPaceAmp input; aPaceWidth input; vPaceWidth input; ARP input; VRP input; lowrateInterval input; a_sense input; v_sense input; mode input; Z_VENT_CTRL output; PACING_REF_PWM output; PACE_GND_CTRL output; FRONTEND_CTRL output; VENT_CMP_REF_PWM output; ATR_CMP_REF_PWM output; hysteresisInterval input; hysteresis input; rate_adapt_interval input

== stateflow chart d2_pacemaker_rate_adaptive/Subsystem3/Chart ==
  state PARAMETER_SETTING
    entry:
    mode=typecast(rxdata(3:4), 'uint16');
    A_pulse_width=typecast(rxdata(5:6),'uint16');
    V_pulse_width=typecast(rxdata(7:8),'uint16');
    lower_rate_limit=typecast(rxdata(9:10),'uint16');
    A_amp=typecast(rxdata(11:14),'single');
    V_amp=typecast(rxdata(15:18),'single');
    A_refractory=typecast(rxdata(19:20),'uint16');
    V_refractory=typecast(rxdata(21:22),'uint16');
    A_or_V_delay=typecast(rxdata(23:24),'uint16');
    A_sensitivity=typecast(rxdata(25:28),'single')/3.3*100;
    V_sensitivity=typecast(rxdata(29:32),'single')/3.3*100;
    recovery_time=typecast(rxdata(33:34),'uint16');
    response_factor=typecast(rxdata(35:36),'uint16');
    max_sensor_rate=typecast(rxdata(37:38),'uint16');
    activity_threshold=typecast(rxdata(39:42),'single');
    reaction_time=typecast(rxdata(43:44),'uint16');
    upper_rate_limit=typecast(rxdata(45:46),'uint16');
  state INITIAL
    entry:
    mode=3;
    lower_rate_limit = 60;
    A_pulse_width = 1;
    V_pulse_width = 1;
    A_amp = 70;
    V_amp = 70
    A_refractory=250;
    V_refractory=320;
    activity_threshold=1.2;
    reaction_time=6;
    A_sensitivity=70;
    V_sensitivity=70;
    A_or_V_delay=150;
    recover_time=12;
    response_factor=10;
    max_sensor_rate=120;
    upper_rate_limit=120;
  state STANDBY
  state SENDING_PARAMS
    entry:
    send_params();
  PARAMETER_SETTING -> SENDING_PARAMS
  (junction 7) -> PARAMETER_SETTING [order 1] : [rxdata(1)==hex2dec('16') && rxdata(2)==hex2dec('55')]
  (default) -> INITIAL
  (junction 7) -> STANDBY [order 3]
  INITIAL -> STANDBY
  STANDBY -> (junction 7) : [status==0]
  (junction 7) -> SENDING_PARAMS [order 2] : [rxdata(1)==hex2dec('16')&&rxdata(2)==hex2dec('22')]
  SENDING_PARAMS -> STANDBY
  data: rxdata input; status input; A_amp output; A_or_V_delay output; A_pulse_width output; A_refractory output; A_sensitivity output; V_amp output; V_pulse_width output; V_refractory output; V_sensitivity output; activity_threshold output; lower_rate_limit output; max_sensor_rate output; mode output; reaction_time output; recover_time output; recovery_time output; response_factor output double; upper_rate_limit output

== stateflow chart d2_pacemaker_rate_adaptive/Subsystem6/Subsystem5/Chart1 ==
  state ACCELERATION
    entry:
    new_pacing_rate = current_pacing_rate + (maximum_sensor_rate - lowRate) / (reaction_time*100)
  state INIT
    entry:
    new_pacing_rate = lowRate;
  state STEADY
    entry:
    new_pacing_rate = current_pacing_rate;
  state DEACCELERATION
    entry:
    new_pacing_rate = current_pacing_rate - (maximum_sensor_rate - lowRate) / (recovery_time*100)
  ACCELERATION -> ACCELERATION [order 3] : after(10,msec)
  (default) -> INIT
  STEADY -> ACCELERATION [order 1] : [desired_pacing_rate>current_pacing_rate]
  ACCELERATION -> STEADY [order 1] : [desired_pacing_rate==current_pacing_rate]
  DEACCELERATION -> ACCELERATION [order 2] : [desired_pacing_rate>current_pacing_rate]
  ACCELERATION -> DEACCELERATION [order 2] : [desired_pacing_rate<current_pacing_rate]
  INIT -> STEADY
  STEADY -> STEADY [order 3] : after(10,msec)
  STEADY -> DEACCELERATION [order 2] : [desired_pacing_rate<current_pacing_rate]
  DEACCELERATION -> STEADY [order 1] : [desired_pacing_rate==current_pacing_rate]
  DEACCELERATION -> DEACCELERATION [order 3] : after(10,msec)
  data: current_pacing_rate input; reaction_time input; recovery_time input; desired_pacing_rate input; lowRate input; maximum_sensor_rate input; new_pacing_rate output
